simulink model "test"  (R2023b)
settings: Solver=FixedStepAuto  StartTime=0  StopTime=5000  FixedStep=0.1  RelTol=1e-3
model workspace: external: MATLAB File par.m (data not in the file)
values from neighbouring files (symbols this model uses):
  K_guiti = 2.4    [par.m]
undefined symbols (not defined in the file or in its folder): T_en
settings Model: Creator=wangxueli  LastModifiedBy=wangxueli

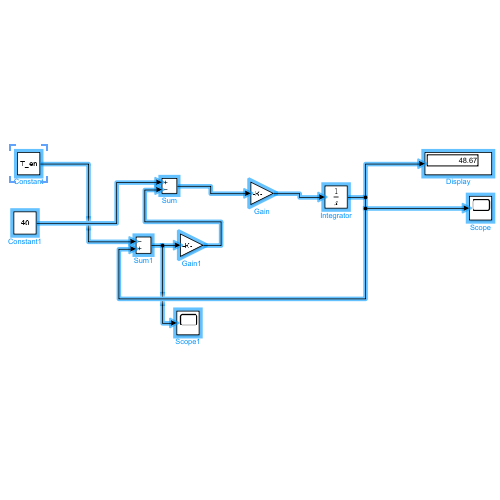
[thumbnail: Simulink's stored preview of the top-level diagram]
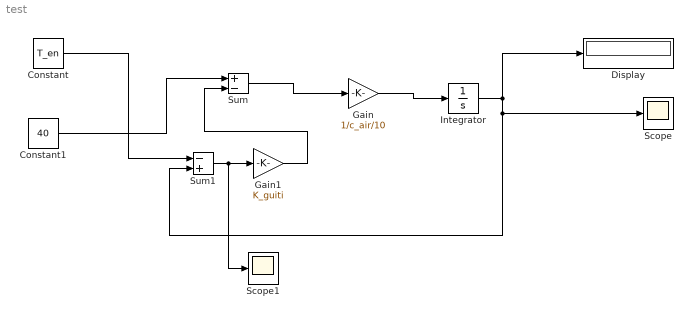
== system test ==
  Constant : Constant  Value=T_en
  Constant1 : Constant  Value=40
  Display : Display
  Gain : Gain  Gain=1/c_air/10
  Gain1 : Gain  Gain=K_guiti
  Integrator : Integrator  InitialCondition=25
  Scope : Scope
  Scope1 : Scope
  Sum : Sum  Inputs=+-
  Sum1 : Sum  Inputs=-+
  wires:
  Sum/1 -> Gain/1
  Gain/1 -> Integrator/1
  Integrator/1 -> Scope/1, Sum1/2, Display/1
  Constant/1 -> Sum1/1
  Sum1/1 -> Scope1/1, Gain1/1
  Gain1/1 -> Sum/2
  Constant1/1 -> Sum/1
